simulink model "GVCU_HIL"  (R2026a)
settings: Solver=ode3  StartTime=0  StopTime=2474  FixedStep=0.0002
model workspace (MAT data in the model file):
  CANoelibParameters : object (value not decoded)
values from neighbouring files (symbols this model uses):
  acc_pedal_data = pedal_data.accelerator_pedal_position_t0    [Vehicle_Simulink_init.m]
  acc_pedal_time = pedal_data.t0    [Vehicle_Simulink_init.m]
  brk_pedal_data = brake_pedal_data.shared_brakes_drvrBrkPedlPerc_t0    [Vehicle_Simulink_init.m]
  brk_pedal_time = brake_pedal_data.t0    [Vehicle_Simulink_init.m]
  cycle_len = zeros(1, num_cycles)    [Vehicle_Simulink_init.m]
  cycle_speed_matrix = zeros(max_cycle_len, num_cycles)    [Vehicle_Simulink_init.m]
  cycle_time_matrix = zeros(max_cycle_len, num_cycles)    [Vehicle_Simulink_init.m]
  veh_speed_data = speed_data.shared_dynamicsVso_vehVelLgt_t0    [Vehicle_Simulink_init.m]
  veh_speed_time = speed_data.t0    [Vehicle_Simulink_init.m]
undefined symbols (not defined in the file or in its folder): Active, AuxActive, bat, environment, FL_prs_voltage, FR_prs_voltage, pos, RL_prs_voltage, RR_prs_voltage, tir, veh, VGetRawValueFlag, Voltage, VT2816_1_Ch1, VT2816_1_Ch2, VT2816_1_Ch3, VT2816_1_Ch4, VT2816_3_Ch13, VT2816_3_Ch14, VT7101_1_Out2, VT7820_2_Channel1, VT7820_2_Channel2, VT7820_2_Channel3, VT7820_2_Channel4, VTS
libraries: canoelib x144, autolibsharedcoupling x21, autolibcoupling x9, autolibshared x5, simulink_extras x4, simulink x4, slpidlib x3, autolibshareddiff x3, autolibutils x1, autolibdatasheetbattery x1, autolibmappedmotor x1, sl_discontinuities x1
(part 9 of 9)

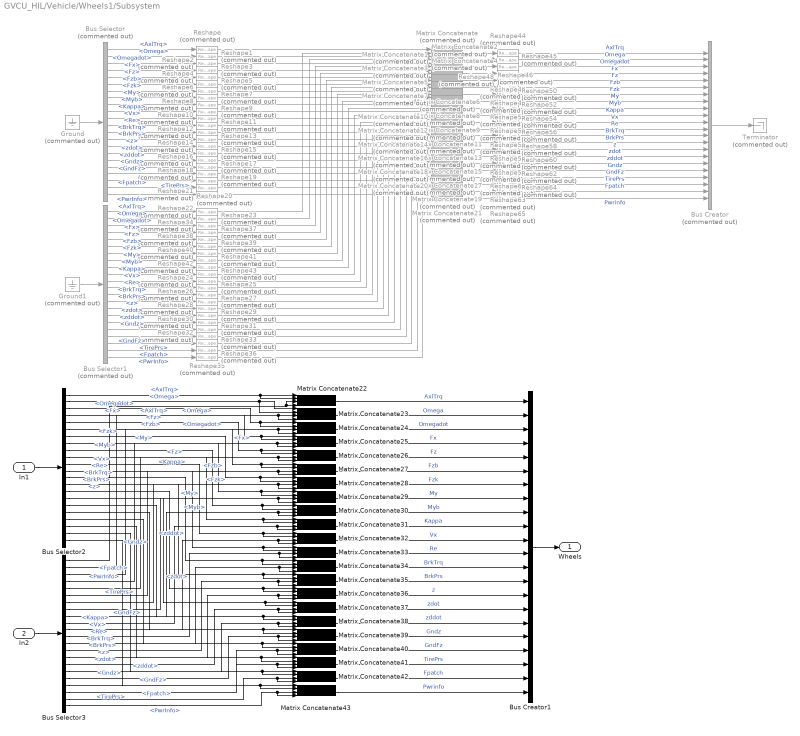
== system GVCU_HIL/Vehicle/Wheels1/Subsystem ==
  In1 : Inport
  In2 : Inport  Port=2
  Bus Creator : BusCreator  Commented=on  Inputs=22
  Bus Creator1 : BusCreator  Inputs=22
  Bus Selector : BusSelector  Commented=on  OutputSignals=AxlTrq,Omega,Omegadot,Fx,Fz,Fzb,Fzk,My,Myb,Kappa,Vx,Re,BrkTrq,BrkPrs,z,zdot,zddot,Gndz,GndFz,TirePrs,Fpatch,PwrInfo
  Bus Selector1 : BusSelector  Commented=on  OutputSignals=AxlTrq,Omega,Omegadot,Fx,Fz,Fzb,Fzk,My,Myb,Kappa,Vx,Re,BrkTrq,BrkPrs,z,zdot,zddot,Gndz,GndFz,TirePrs,Fpatch,PwrInfo
  Bus Selector2 : BusSelector  OutputSignals=AxlTrq,Omega,Omegadot,Fx,Fz,Fzb,Fzk,My,Myb,Kappa,Vx,Re,BrkTrq,BrkPrs,z,zdot,zddot,Gndz,GndFz,TirePrs,Fpatch,PwrInfo
  Bus Selector3 : BusSelector  OutputSignals=AxlTrq,Omega,Omegadot,Fx,Fz,Fzb,Fzk,My,Myb,Kappa,Vx,Re,BrkTrq,BrkPrs,z,zdot,zddot,Gndz,GndFz,TirePrs,Fpatch,PwrInfo
  Ground : Ground  Commented=on
  Ground1 : Ground  Commented=on
  Matrix Concatenate : Concatenate  Commented=on
  Matrix Concatenate{1..21} (21 alike) : Concatenate  Commented=on  ConcatenateDimension=2
  Matrix Concatenate{22..43} (22 alike) : Concatenate  NumInputs=4
  Reshape{,1..43} (44 alike) : Reshape  Commented=on  OutputDimensionality=Row vector (2-D)
  Reshape{44..65} (22 alike) : Reshape  Commented=on
  Terminator : Terminator  Commented=on
  Wheels : Outport
  wires:
  Bus Selector/1 -> Reshape/1  "<AxlTrq>"
  In2/1 -> Bus Selector3/1
  In1/1 -> Bus Selector2/1
  Bus Selector3/22 -> Matrix Concatenate43/3, Matrix Concatenate43/4  "<PwrInfo>"
  Bus Selector3/21 -> Matrix Concatenate42/3, Matrix Concatenate42/4  "<Fpatch>"
  Bus Selector3/20 -> Matrix Concatenate41/3, Matrix Concatenate41/4  "<TirePrs>"
  Bus Selector3/19 -> Matrix Concatenate40/3, Matrix Concatenate40/4  "<GndFz>"
  Bus Selector3/18 -> Matrix Concatenate39/3, Matrix Concatenate39/4  "<Gndz>"
  Bus Selector3/17 -> Matrix Concatenate38/3, Matrix Concatenate38/4  "<zddot>"
  Bus Selector3/16 -> Matrix Concatenate37/3, Matrix Concatenate37/4  "<zdot>"
  Bus Selector3/15 -> Matrix Concatenate36/3, Matrix Concatenate36/4  "<z>"
  Bus Selector3/14 -> Matrix Concatenate35/3, Matrix Concatenate35/4  "<BrkPrs>"
  Bus Selector3/13 -> Matrix Concatenate34/3, Matrix Concatenate34/4  "<BrkTrq>"
  Bus Selector3/12 -> Matrix Concatenate33/3, Matrix Concatenate33/4  "<Re>"
  Bus Selector3/11 -> Matrix Concatenate32/3, Matrix Concatenate32/4  "<Vx>"
  Bus Selector3/10 -> Matrix Concatenate31/3, Matrix Concatenate31/4  "<Kappa>"
  Bus Selector3/9 -> Matrix Concatenate30/3, Matrix Concatenate30/4  "<Myb>"
  Bus Selector3/8 -> Matrix Concatenate29/3, Matrix Concatenate29/4  "<My>"
  Bus Selector3/7 -> Matrix Concatenate28/3, Matrix Concatenate28/4  "<Fzk>"
  Bus Selector3/6 -> Matrix Concatenate27/3, Matrix Concatenate27/4  "<Fzb>"
  Bus Selector3/5 -> Matrix Concatenate26/3, Matrix Concatenate26/4  "<Fz>"
  Bus Selector3/4 -> Matrix Concatenate25/3, Matrix Concatenate25/4  "<Fx>"
  Bus Selector3/3 -> Matrix Concatenate24/3, Matrix Concatenate24/4  "<Omegadot>"
  Bus Selector3/2 -> Matrix Concatenate23/3, Matrix Concatenate23/4  "<Omega>"
  Bus Selector3/1 -> Matrix Concatenate22/3, Matrix Concatenate22/4  "<AxlTrq>"
  Matrix Concatenate23/1 -> Bus Creator1/2  "Omega"
  Matrix Concatenate29/1 -> Bus Creator1/8  "My"
  Matrix Concatenate36/1 -> Bus Creator1/15  "z"
  Matrix Concatenate27/1 -> Bus Creator1/6  "Fzb"
  Matrix Concatenate25/1 -> Bus Creator1/4  "Fx"
  Matrix Concatenate33/1 -> Bus Creator1/12  "Re"
  Matrix Concatenate28/1 -> Bus Creator1/7  "Fzk"
  Matrix Concatenate30/1 -> Bus Creator1/9  "Myb"
  Matrix Concatenate31/1 -> Bus Creator1/10  "Kappa"
  Matrix Concatenate43/1 -> Bus Creator1/22  "Pwrinfo"
  Matrix Concatenate22/1 -> Bus Creator1/1  "AxlTrq"
  Matrix Concatenate38/1 -> Bus Creator1/17  "zddot"
  Matrix Concatenate37/1 -> Bus Creator1/16  "zdot"
  Matrix Concatenate41/1 -> Bus Creator1/20  "TirePrs"
  Matrix Concatenate39/1 -> Bus Creator1/18  "Gndz"
  Matrix Concatenate24/1 -> Bus Creator1/3  "Omegadot"
  Matrix Concatenate26/1 -> Bus Creator1/5  "Fz"
  Matrix Concatenate35/1 -> Bus Creator1/14  "BrkPrs"
  Matrix Concatenate42/1 -> Bus Creator1/21  "Fpatch"
  Matrix Concatenate40/1 -> Bus Creator1/19  "GndFz"
  Matrix Concatenate34/1 -> Bus Creator1/13  "BrkTrq"
  Matrix Concatenate32/1 -> Bus Creator1/11  "Vx"
  Bus Creator1/1 -> Wheels/1
  Bus Selector2/22 -> Matrix Concatenate43/2, Matrix Concatenate43/1  "<PwrInfo>"
  Bus Selector2/21 -> Matrix Concatenate42/1, Matrix Concatenate42/2  "<Fpatch>"
  Bus Selector2/20 -> Matrix Concatenate41/1, Matrix Concatenate41/2  "<TirePrs>"
  Bus Selector2/19 -> Matrix Concatenate40/1, Matrix Concatenate40/2  "<GndFz>"
  Bus Selector2/18 -> Matrix Concatenate39/1, Matrix Concatenate39/2  "<Gndz>"
  Bus Selector2/17 -> Matrix Concatenate38/1, Matrix Concatenate38/2  "<zddot>"
  Bus Selector2/16 -> Matrix Concatenate37/1, Matrix Concatenate37/2  "<zdot>"
  Bus Selector2/15 -> Matrix Concatenate36/1, Matrix Concatenate36/2  "<z>"
  Bus Selector2/14 -> Matrix Concatenate35/1, Matrix Concatenate35/2  "<BrkPrs>"
  Bus Selector2/13 -> Matrix Concatenate34/2, Matrix Concatenate34/1  "<BrkTrq>"
  Bus Selector2/12 -> Matrix Concatenate33/1, Matrix Concatenate33/2  "<Re>"
  Bus Selector2/11 -> Matrix Concatenate32/2, Matrix Concatenate32/1  "<Vx>"
  Bus Selector2/10 -> Matrix Concatenate31/1, Matrix Concatenate31/2  "<Kappa>"
  Bus Selector2/9 -> Matrix Concatenate30/1, Matrix Concatenate30/2  "<Myb>"
  Bus Selector2/8 -> Matrix Concatenate29/1, Matrix Concatenate29/2  "<My>"
  Bus Selector2/7 -> Matrix Concatenate28/1, Matrix Concatenate28/2  "<Fzk>"
  Bus Selector2/6 -> Matrix Concatenate27/1, Matrix Concatenate27/2  "<Fzb>"
  Bus Selector2/5 -> Matrix Concatenate26/1, Matrix Concatenate26/2  "<Fz>"
  Bus Selector2/4 -> Matrix Concatenate25/1, Matrix Concatenate25/2  "<Fx>"
  Bus Selector2/3 -> Matrix Concatenate24/2, Matrix Concatenate24/1  "<Omegadot>"
  Bus Selector2/2 -> Matrix Concatenate23/2, Matrix Concatenate23/1  "<Omega>"
  Bus Selector2/1 -> Matrix Concatenate22/1, Matrix Concatenate22/2  "<AxlTrq>"
  Bus Creator/1 -> Terminator/1
  Reshape56/1 -> Bus Creator/13  "BrkTrq"
  Reshape54/1 -> Bus Creator/11  "Vx"
  Reshape55/1 -> Bus Creator/12  "Re"
  Reshape57/1 -> Bus Creator/14  "BrkPrs"
  Reshape58/1 -> Bus Creator/15  "z"
  Reshape59/1 -> Bus Creator/16  "zdot"
  Reshape60/1 -> Bus Creator/17  "zddot"
  Reshape61/1 -> Bus Creator/18  "Gndz"
  Reshape62/1 -> Bus Creator/19  "GndFz"
  Reshape63/1 -> Bus Creator/20  "TirePrs"
  Reshape64/1 -> Bus Creator/21  "Fpatch"
  Reshape65/1 -> Bus Creator/22  "Pwrinfo"
  Reshape53/1 -> Bus Creator/10  "Kappa"
  Reshape52/1 -> Bus Creator/9  "Myb"
  Reshape51/1 -> Bus Creator/8  "My"
  Reshape50/1 -> Bus Creator/7  "Fzk"
  Reshape49/1 -> Bus Creator/6  "Fzb"
  Reshape48/1 -> Bus Creator/5  "Fz"
  Reshape47/1 -> Bus Creator/4  "Fx"
  Reshape46/1 -> Bus Creator/3  "Omegadot"
  Reshape45/1 -> Bus Creator/2  "Omega"
  Reshape44/1 -> Bus Creator/1  "AxlTrq"
  Matrix Concatenate21/1 -> Reshape65/1
  Matrix Concatenate20/1 -> Reshape64/1
  Matrix Concatenate19/1 -> Reshape63/1
  Matrix Concatenate18/1 -> Reshape62/1
  Matrix Concatenate17/1 -> Reshape61/1
  Matrix Concatenate16/1 -> Reshape60/1
  Matrix Concatenate15/1 -> Reshape59/1
  Matrix Concatenate14/1 -> Reshape58/1
  Matrix Concatenate13/1 -> Reshape57/1
  Matrix Concatenate12/1 -> Reshape56/1
  Matrix Concatenate11/1 -> Reshape55/1
  Matrix Concatenate10/1 -> Reshape54/1
  Matrix Concatenate9/1 -> Reshape53/1
  Matrix Concatenate8/1 -> Reshape52/1
  Matrix Concatenate7/1 -> Reshape51/1
  Matrix Concatenate6/1 -> Reshape50/1
  Matrix Concatenate5/1 -> Reshape49/1
  Matrix Concatenate4/1 -> Reshape48/1
  Matrix Concatenate3/1 -> Reshape47/1
  Matrix Concatenate2/1 -> Reshape46/1
  Matrix Concatenate1/1 -> Reshape45/1
  Matrix Concatenate/1 -> Reshape44/1
  Reshape25/1 -> Matrix Concatenate11/2
  Reshape26/1 -> Matrix Concatenate12/2
  Reshape27/1 -> Matrix Concatenate13/2
  Reshape28/1 -> Matrix Concatenate14/2
  Reshape29/1 -> Matrix Concatenate15/2
  Reshape30/1 -> Matrix Concatenate16/2
  Reshape31/1 -> Matrix Concatenate17/2
  Reshape32/1 -> Matrix Concatenate18/2
  Reshape33/1 -> Matrix Concatenate19/2
  Reshape35/1 -> Matrix Concatenate20/2
  Reshape36/1 -> Matrix Concatenate21/2
  Reshape24/1 -> Matrix Concatenate10/2
  Reshape43/1 -> Matrix Concatenate9/2
  Reshape42/1 -> Matrix Concatenate8/2
  Reshape41/1 -> Matrix Concatenate7/2
  Reshape40/1 -> Matrix Concatenate6/2
  Reshape39/1 -> Matrix Concatenate5/2
  Reshape21/1 -> Matrix Concatenate21/1
  Reshape20/1 -> Matrix Concatenate20/1
  Reshape19/1 -> Matrix Concatenate19/1
  Reshape18/1 -> Matrix Concatenate18/1
  Reshape17/1 -> Matrix Concatenate17/1
  Reshape16/1 -> Matrix Concatenate16/1
  Reshape15/1 -> Matrix Concatenate15/1
  Reshape14/1 -> Matrix Concatenate14/1
  Reshape13/1 -> Matrix Concatenate13/1
  Reshape12/1 -> Matrix Concatenate12/1
  Reshape11/1 -> Matrix Concatenate11/1
  Reshape10/1 -> Matrix Concatenate10/1
  Reshape9/1 -> Matrix Concatenate9/1
  Reshape8/1 -> Matrix Concatenate8/1
  Reshape7/1 -> Matrix Concatenate7/1
  Reshape6/1 -> Matrix Concatenate6/1
  Reshape5/1 -> Matrix Concatenate5/1
  Reshape38/1 -> Matrix Concatenate4/2
  Reshape37/1 -> Matrix Concatenate3/2
  Reshape4/1 -> Matrix Concatenate4/1
  Reshape3/1 -> Matrix Concatenate3/1
  Reshape34/1 -> Matrix Concatenate2/2
  Reshape2/1 -> Matrix Concatenate2/1
  Reshape23/1 -> Matrix Concatenate1/2
  Reshape1/1 -> Matrix Concatenate1/1
  Reshape22/1 -> Matrix Concatenate/2
  Reshape/1 -> Matrix Concatenate/1
  Bus Selector1/19 -> Reshape32/1  "<GndFz>"
  Bus Selector1/13 -> Reshape26/1  "<BrkTrq>"
  Bus Selector1/15 -> Reshape28/1  "<z>"
  Bus Selector1/5 -> Reshape38/1  "<Fz>"
  Ground1/1 -> Bus Selector1/1
  Bus Selector1/14 -> Reshape27/1  "<BrkPrs>"
  Bus Selector1/1 -> Reshape22/1  "<AxlTrq>"
  Bus Selector1/10 -> Reshape43/1  "<Kappa>"
  Bus Selector1/6 -> Reshape39/1  "<Fzb>"
  Bus Selector1/11 -> Reshape24/1  "<Vx>"
  Bus Selector1/18 -> Reshape31/1  "<Gndz>"
  Bus Selector1/8 -> Reshape41/1  "<My>"
  Bus Selector1/22 -> Reshape36/1  "<PwrInfo>"
  Bus Selector1/21 -> Reshape35/1  "<Fpatch>"
  Bus Selector1/17 -> Reshape30/1  "<zddot>"
  Bus Selector1/2 -> Reshape23/1  "<Omega>"
  Bus Selector1/12 -> Reshape25/1  "<Re>"
  Bus Selector1/20 -> Reshape33/1  "<TirePrs>"
  Bus Selector1/9 -> Reshape42/1  "<Myb>"
  Bus Selector1/16 -> Reshape29/1  "<zdot>"
  Bus Selector1/7 -> Reshape40/1  "<Fzk>"
  Bus Selector1/3 -> Reshape34/1  "<Omegadot>"
  Bus Selector1/4 -> Reshape37/1  "<Fx>"
  Bus Selector/22 -> Reshape21/1  "<PwrInfo>"
  Bus Selector/21 -> Reshape20/1  "<Fpatch>"
  Bus Selector/20 -> Reshape19/1  "<TirePrs>"
  Bus Selector/19 -> Reshape18/1  "<GndFz>"
  Bus Selector/18 -> Reshape17/1  "<Gndz>"
  Bus Selector/17 -> Reshape16/1  "<zddot>"
  Bus Selector/16 -> Reshape15/1  "<zdot>"
  Bus Selector/15 -> Reshape14/1  "<z>"
  Bus Selector/14 -> Reshape13/1  "<BrkPrs>"
  Bus Selector/13 -> Reshape12/1  "<BrkTrq>"
  Bus Selector/12 -> Reshape11/1  "<Re>"
  Bus Selector/11 -> Reshape10/1  "<Vx>"
  Bus Selector/10 -> Reshape9/1  "<Kappa>"
  Bus Selector/9 -> Reshape8/1  "<Myb>"
  Bus Selector/8 -> Reshape7/1  "<My>"
  Bus Selector/7 -> Reshape6/1  "<Fzk>"
  Bus Selector/6 -> Reshape5/1  "<Fzb>"
  Bus Selector/5 -> Reshape4/1  "<Fz>"
  Bus Selector/4 -> Reshape3/1  "<Fx>"
  Bus Selector/3 -> Reshape2/1  "<Omegadot>"
  Bus Selector/2 -> Reshape1/1  "<Omega>"
  Ground/1 -> Bus Selector/1

== system GVCU_HIL/Vehicle/Wheels1/whel to axel transform3 ==
  Input (1x4) : Inport
  Selector4 : Selector  InputPortWidth=4  IndexOptions=Index vector (dialog)  Indices=[1]  OutputSizes=1
  Selector5 : Selector  InputPortWidth=4  IndexOptions=Index vector (dialog)  Indices=[2]  OutputSizes=1
  Selector6 : Selector  InputPortWidth=4  IndexOptions=Index vector (dialog)  Indices=[3]  OutputSizes=1
  Selector7 : Selector  InputPortWidth=4  IndexOptions=Index vector (dialog)  Indices=[4]  OutputSizes=1
  "Front L " : Outport
  Front R : Outport  Port=2
  "Rear L " : Outport  Port=3
  Rear R : Outport  Port=4
  wires:
  Selector7/1 -> Rear R/1
  Selector6/1 -> "Rear L "/1
  Selector5/1 -> Front R/1
  Selector4/1 -> "Front L "/1
  Input (1x4)/1 -> Selector4/1, Selector5/1, Selector7/1, Selector6/1

== matlab function GVCU_HIL/Clutch handling/Offset_substraction/MATLAB Function ==
  data: drvMode input; y output; pPa input
function y = fcn(drvMode, pPa)
% drvMode : drive mode input
% pPa     : measured pressure input in Pa
% y       : pressure output with learned offset removed, in Pa

persistent prevDrvMode state timer sumP sampleCount offset

if isempty(prevDrvMode)
    prevDrvMode = drvMode;
    state = uint8(0);      % 0=idle, 1=wait, 2=average, 3=hold
    timer = 0.0;
    sumP = 0.0;
    sampleCount = uint32(0);
    offset = 0.0;
end

T = 0.0002;          % sample time [s]
WAIT_TIME = 0.5;     % wait time after drvMode becomes 1 [s]
AVG_TIME  = 0.2;     % averaging time [s]
ONE_BAR_PA = 1e5;    % 1 bar in Pa

% Trigger when drvMode becomes 1, regardless of previous value
if (prevDrvMode ~= 1) && (drvMode == 1)
    state = uint8(1);
    timer = 0.0;
    sumP = 0.0;
    sampleCount = uint32(0);
end

switch state
    case 0
        % Idle state

    case 1
        % Wait for 0.5 s
        timer = timer + T;
        if timer >= WAIT_TIME
            state = uint8(2);
            timer = 0.0;
            sumP = 0.0;
            sampleCount = uint32(0);
        end

    case 2
        % Average pressure for 0.2 s
        timer = timer + T;
        sumP = sumP + pPa;
        sampleCount = sampleCount + 1;

        if timer >= AVG_TIME
            if sampleCount > 0
                offset = sumP / double(sampleCount) - ONE_BAR_PA;
            else
                offset = 0.0;
            end
            state = uint8(3);
        end

    case 3
        % Hold learned offset
end

% Output compensated pressure
y = pPa - offset;

prevDrvMode = drvMode;

== matlab function GVCU_HIL/Powertrain (EV)/PID Speed Ctrl Mode/MATLAB Function1 ==
  settings: updateMethod=DISCRETE
  data: spdErr_rads input; trq_cmd output; trq_fwd input; trq_act input; lim_pos input; lim_neg input; reset input
function trq_cmd = speedPID(spdErr_rads, trq_fwd, trq_act, lim_pos, lim_neg, reset)
%#codegen
% Speed PID + feedforward, output clamped.
% Replicates inverter torque_handler.c trqHandlerSpeedCtrl()
%
% Inputs:
%   spdErr_rads  [rad/s]   speed error (spd_req - spd_fb), computed externally
%   trq_fwd      [Nm]      feedforward torque = GVCU torque request (added internally)
%   trq_act      [Nm]      actual motor torque feedback (e.g. EM_trq from motor model)
%   lim_pos      [Nm]      upper output clamp
%   lim_neg      [Nm]      lower output clamp
%   reset                  from spdCtrlReset block (>0.5 = active)
%
% Output:
%   trq_cmd  [Nm]      clamped torque command (PID + feedforward)
%
% Gains (caldata.c index 0, RPM-based, Ts=500us):
%   kp=2.5, ki=0.004, kaw=0.0035, kd=0

persistent intgl trqReqPrev

if isempty(intgl)
    intgl      = 0;
    trqReqPrev = 0;
end

Ts      = 0.0002;       % actual Simulink step size
Ts_inv  = 0.0005;       % inverter design step size
scale   = Ts / Ts_inv;  % = 0.4

% values from Set 3 
kp  = 2; %0.78;
ki  = 0.035 * scale;    % = 0.0016
kaw = 0.005 * scale;   % = 0.0014

if reset > 0.5
    intgl      = 0;
    trqReqPrev = 0;
    trq_cmd    = 0;
    return;
end

% Speed error in RPM (matches inverter: spdErr = spdReq - ctrlOutSpeed)
spdErr = spdErr_rads * (60 / (2*pi));

% Integrator update with anti-windup
% Matches inverter: spdIntgl += ki*spdErr + kaw*(trqAct - trqReq_prev_unclamped)
intgl = intgl + ki * spdErr + kaw * (trq_act - trqReqPrev);

% Unclamped total output (PID + feedforward)
trq_req_unc = kp * spdErr + intgl + trq_fwd;

% Clamp output
trq_cmd = max(lim_neg, min(lim_pos, trq_req_unc));

% Store unclamped total for next step's anti-windup
trqReqPrev = trq_cmd;

== matlab function GVCU_HIL/Brake_HIL/Simulated GVCU - Steering /MATLAB Function1 ==
  settings: updateMethod=DISCRETE  sampleTime=0.1
  data: y output
function y = counterFcn()
    persistent count;
    if isempty(count)
        count = 0; % Initialize counter
    end
    count = mod(count + 1, 15); % 4-bit counter (0-15)
    y = count; % Use uint8 to avoid Fixed-Point Designer
end

== matlab function GVCU_HIL/Powertrain (EV)/PID Speed Controller/MATLAB Function ==
  settings: updateMethod=DISCRETE
  data: EM_Spd input; reset_out output; speed_req input; t input
function reset_out = spdCtrlReset(EM_Spd, speed_req, t)
% Resets PID integrator when both speeds are below threshold for 500ms.
% Matches real inverter: cInvStopSpeed = 20 RPM, SPD_CTRL_RESET_DELAY = 500ms
% Input t: simulation time from Clock block [s]

persistent stop_ts fired

if isempty(stop_ts)
    stop_ts = 0;
    fired   = false;
end

SPD_THRESHOLD  = 2.094;  % 20 RPM in rad/s  (= cInvStopSpeed)
RESET_DELAY_S  = 0.5;    % 500ms in s       (= SPD_CTRL_RESET_DELAY)

if (abs(EM_Spd) < SPD_THRESHOLD) && (abs(speed_req) < SPD_THRESHOLD)
    if stop_ts == 0
        stop_ts = t;     % Start timer: record entry time
    end

    if ((t - stop_ts) >= RESET_DELAY_S) && (~fired)
        reset_out = 1.0; % Rising edge -> reset PID integrator
        fired     = true;
    else
        reset_out = 0.0;
    end
else
    stop_ts   = 0;       % Reset timer
    fired     = false;   % Allow trigger again next standstill
    reset_out = 0.0;
end

== matlab function GVCU_HIL/Brake_HIL/Simulated GVCU - Steering /MATLAB Function2 ==
  data: switch_state input; drv_st output
function drv_st   = update_drv_st(switch_state)
    % Persistent variables to maintain state across function calls
    persistent drv_st_internal last_switch_state last_update_time;
    
    if isempty(drv_st_internal)
        drv_st_internal = 1;  % Initial state of drv_st
        last_switch_state = 0; % Initial switch state
        last_update_time = tic; % Start timer
    end
    
    if switch_state == 1
        
        if last_switch_state == 0
            % Switch was just turned ON, reset timer and set drv_st to 1
            drv_st_internal = 1;
            last_update_time = tic;
        else
            % Check elapsed time since last update
            elapsed_time = toc(last_update_time);
            if drv_st_internal == 1 && elapsed_time >= 2
                drv_st_internal = 2;
                last_update_time = tic;
            elseif drv_st_internal == 2 && elapsed_time >= 2
                drv_st_internal = 4;
                last_update_time = tic;
            end
        end
        
    else
        
        drv_st_internal = 1; % Reset drv_st if switch is OFF
    end
    
    last_switch_state = switch_state; % Update switch state memory
    drv_st = drv_st_internal; % Output the updated drv_st value
end

== matlab function GVCU_HIL/Brake_HIL/Simulated GVCU - Steering /MATLAB Function3 ==
  settings: updateMethod=DISCRETE  sampleTime=0.01
  data: y output
function y = counterFcn()
    persistent count;
    if isempty(count)
        count = 0; % Initialize counter
    end
    count = mod(count + 1, 15); % 4-bit counter (0-15)
    y = count; % Use uint8 to avoid Fixed-Point Designer
end

== matlab function GVCU_HIL/Brake_HIL/Simulated GVCU - Steering /MATLAB Function4 ==
  settings: updateMethod=DISCRETE  sampleTime=0.01
  data: y output
function y = counterFcn()
    persistent count;
    if isempty(count)
        count = 0; % Initialize counter
    end
    count = mod(count + 1, 15); % 4-bit counter (0-15)
    y = count; % Use uint8 to avoid Fixed-Point Designer
end

== matlab function GVCU_HIL/Brake_HIL/Simulated GVCU - Steering /MATLAB Function5 ==
  settings: updateMethod=DISCRETE  sampleTime=0.1
  data: y output
function y = counterFcn()
    persistent count;
    if isempty(count)
        count = 0; % Initialize counter
    end
    count = mod(count + 1, 15); % 4-bit counter (0-15)
    y = count; % Use uint8 to avoid Fixed-Point Designer
end

== matlab function GVCU_HIL/Inverter/INV ==
  data: inv_st_prev input; inv_st output; inv_ena_req input; motor_ena_req input; inv_shutdown_req input
function inv_st = fcn(inv_st_prev, inv_ena_req, motor_ena_req, inv_shutdown_req)
	switch inv_st_prev
		case 0
			if (1 == inv_ena_req)
				inv_st_local = 1;
			else
				inv_st_local = 0;
			end
		case 1
			if (1 == inv_ena_req)
				inv_st_local = 2;
			else
				inv_st_local = 0;
			end	
		case 2
			if (1 == inv_ena_req)
				inv_st_local = 3;
			else
				inv_st_local = 0;
			end
		case 3
			if ((1 == inv_ena_req) && (1 == motor_ena_req))
				inv_st_local = 4;
			else
				inv_st_local = 3;
			end
		case 4
			if ((1 ~= inv_ena_req) || (1 ~= motor_ena_req) || (1 == inv_shutdown_req))
				inv_st_local = 0;
			else
				inv_st_local = 4;
			end
		case 5
			inv_st_local = 0;
		case 6
			inv_st_local = 0;
		otherwise
			inv_st_local = 0;
	end
	inv_st = inv_st_local;
 
end

== matlab function GVCU_HIL/GVCU - HiL/BMS ==
  data: bms_st_prev input; pwr_st input; bms_st output; hyb_st input
function bms_st = fcn(bms_st_prev, pwr_st, hyb_st)
	switch bms_st_prev
		case 0
			bms_st_local = 5;
		case 1
			if (7 ~= pwr_st)
				bms_st_local = 5;
            elseif (4 == hyb_st)
				bms_st_local = 3;
			else
				bms_st_local = 1;
			end	
		case 2
			bms_st_local = 5;
		case 3
			if (7 ~= pwr_st)
				bms_st_local = 5;
			else
				bms_st_local = 3;
			end
		case 4
			bms_st_local = 5;
		case 5
			if (7 == pwr_st)
				bms_st_local = 3;
			else
				bms_st_local = 5;
			end
		case 6
			bms_st_local = 5;
		otherwise
			bms_st_local = 5;
	end
    bms_st = bms_st_local;
end

== matlab function GVCU_HIL/Wheel_rates/MATLAB Function2 ==
  data: wheel_rate input; wheel_direction output
function wheel_direction = wheel_direction(wheel_rate)

STATIONARY_THD = 0.01; % rad/s
 
if abs(wheel_rate) <= STATIONARY_THD

    wheel_direction = 2; % STATIONARY

elseif wheel_rate > STATIONARY_THD

    wheel_direction = 3; % FORWARD

elseif wheel_rate < -STATIONARY_THD

    wheel_direction = 4; % REARWARD

else

    wheel_direction = 0; % UNKNOWN (NaN)

end

== matlab function GVCU_HIL/Driver/MATLAB Function ==
  settings: updateMethod=DISCRETE
  data: t_sim input; input_mode input; t_spd input; spd_data input; cycle_idx input; cycle_time_matrix input; cycle_speed_matrix input; cycle_len input; vel_ref input; vel_out output; cycle_time_remaining output; cycle_finished output
function [vel_out, cycle_time_remaining, cycle_finished] = fcn(t_sim, input_mode, t_spd, spd_data, ...
                                                              cycle_idx, cycle_time_matrix, cycle_speed_matrix, cycle_len, vel_ref)

persistent t_mode_start last_mode last_cycle;

if isempty(t_mode_start)
    t_mode_start = -1;
    last_mode    = 0;
    last_cycle   = 0;
end

% Default: WLTC3b
default_cycle_idx = 4;

% Safe cycle index
idx = round(cycle_idx);

if isnan(idx) || idx < 1 || idx > size(cycle_time_matrix, 2)
    idx = default_cycle_idx;
end

% Restart timing when mode changes to replay modes
if (input_mode == 2 || input_mode == 3) && last_mode ~= input_mode
    t_mode_start = t_sim;
end

% Restart drive cycle when selected cycle changes while input_mode == 3
if input_mode == 3 && last_cycle ~= idx
    t_mode_start = t_sim;
end

last_mode  = input_mode;
last_cycle = idx;

% Default outputs
vel_out              = vel_ref;
cycle_time_remaining = 0;
cycle_finished       = 0;

if input_mode == 2 && t_mode_start >= 0

    % Recorded speed replay
    t_rel = t_sim - t_mode_start;
    t_rel = min(t_rel, t_spd(end));

    vel_out = interp1(t_spd, spd_data, t_rel, 'linear', spd_data(end));

elseif input_mode == 3 && t_mode_start >= 0

    % Drive cycle replay
    n = int32(cycle_len(idx));

    cycle_end_time = cycle_time_matrix(n, idx);

    t_rel = t_sim - t_mode_start;

    % Remaining time of selected cycle
    cycle_time_remaining = max(cycle_end_time - t_rel, 0);

    if t_rel >= cycle_end_time
        cycle_finished = 1;
        t_rel = cycle_end_time;
    end

    cycle_time  = cycle_time_matrix(1:n, idx);
    cycle_speed = cycle_speed_matrix(1:n, idx);

    vel_out = interp1(cycle_time, cycle_speed, t_rel, 'linear', cycle_speed(end));

end

== matlab function GVCU_HIL/Driver/MATLAB Function2 ==
  settings: updateMethod=DISCRETE
  data: RefVel input; RefVel output; trans_park_neutral input; ign output; brake_switch output; btn_paddle_ri output; btn_paddle_le output; trans_neutral_drive input; trans_park_drive input
function [RefVel, ign, brake_switch, btn_paddle_ri, btn_paddle_le] = update_drv_st(RefVel, trans_park_neutral, trans_neutral_drive, trans_park_drive)
persistent main_state sub_state t_start
persistent brake_switch_internal
persistent btn_paddle_ri_internal btn_paddle_le_internal
persistent prev_trans_park_neutral prev_trans_neutral_drive prev_trans_park_drive
persistent pending_park_neutral pending_neutral_drive pending_park_drive

% main_state:
% 0 = idle
% 1 = Park -> Neutral
% 2 = Neutral -> Drive
% 3 = Park -> Drive
%
% signal convention:
% brake_switch: 1 = released, 2 = pressed
% btn_paddle_ri: 1 = released, 2 = pressed
% btn_paddle_le: 1 = released, 2 = pressed

if isempty(main_state)
    main_state = 0;
    sub_state = 0;
    t_start = tic;

    brake_switch_internal = 1;
    btn_paddle_ri_internal = 1;
    btn_paddle_le_internal = 1;

    prev_trans_park_neutral = 0;
    prev_trans_neutral_drive = 0;
    prev_trans_park_drive = 0;

    pending_park_neutral = 0;
    pending_neutral_drive = 0;
    pending_park_drive = 0;
end

ign = 7;
refVelInp = RefVel;

% Capture button rising edges and store as one-shot pending requests.
if trans_park_neutral && ~prev_trans_park_neutral
    pending_park_neutral = 1;
end
if trans_neutral_drive && ~prev_trans_neutral_drive
    pending_neutral_drive = 1;
end
if trans_park_drive && ~prev_trans_park_drive
    pending_park_drive = 1;
end

prev_trans_park_neutral = trans_park_neutral;
prev_trans_neutral_drive = trans_neutral_drive;
prev_trans_park_drive = trans_park_drive;

% Only start a new transition when no other transition is active
if main_state == 0
    if pending_park_drive
        main_state = 3;
        sub_state = 0;
        t_start = tic;
        pending_park_drive = 0;

    elseif pending_park_neutral
        main_state = 1;
        sub_state = 0;
        t_start = tic;
        pending_park_neutral = 0;

    elseif pending_neutral_drive
        main_state = 2;
        sub_state = 0;
        t_start = tic;
        pending_neutral_drive = 0;
    end
end

switch main_state
    case 0
        % Idle:
        % keep RefVel input
        % release buttons and brake
        RefVel = refVelInp;
        brake_switch_internal = 1;
        btn_paddle_ri_internal = 1;
        btn_paddle_le_internal = 1;

    case 1
        % Park -> Neutral
        % RefVel forced to zero during transition
        RefVel = 0;

        switch sub_state
            case 0
                % Press brake first
                brake_switch_internal = 2;
                btn_paddle_ri_internal = 1;
                btn_paddle_le_internal = 1;

                sub_state = 1;
                t_start = tic;

            case 1
                % Press both paddles for 1 second
                brake_switch_internal = 2;
                btn_paddle_ri_internal = 2;
                btn_paddle_le_internal = 2;

                if toc(t_start) >= 1.0
                    sub_state = 2;
                    t_start = tic;
                end

            case 2
                % Release both paddles, keep brake pressed
                brake_switch_internal = 2;
                btn_paddle_ri_internal = 1;
                btn_paddle_le_internal = 1;

                if toc(t_start) >= 0.2
                    sub_state = 3;
                end

            case 3
                % Finish in Neutral, then return to idle
                brake_switch_internal = 1;
                btn_paddle_ri_internal = 1;
                btn_paddle_le_internal = 1;

                main_state = 0;
                sub_state = 0;
        end

    case 2
        % Neutral -> Drive
        % RefVel forced to zero during transition
        RefVel = 0;

        switch sub_state
            case 0
                % Press brake first
                brake_switch_internal = 2;
                btn_paddle_ri_internal = 1;
                btn_paddle_le_internal = 1;

                sub_state = 1;
                t_start = tic;

            case 1
                % Press right paddle for 1 second
                brake_switch_internal = 2;
                btn_paddle_ri_internal = 2;
                btn_paddle_le_internal = 1;

                if toc(t_start) >= 1.0
                    sub_state = 2;
                    t_start = tic;
                end

            case 2
                % Release right paddle, keep brake pressed
                brake_switch_internal = 2;
                btn_paddle_ri_internal = 1;
                btn_paddle_le_internal = 1;

                if toc(t_start) >= 0.2
                    sub_state = 3;
                end

            case 3
                % Release brake after paddle release
                brake_switch_internal = 1;
                btn_paddle_ri_internal = 1;
                btn_paddle_le_internal = 1;

                main_state = 0;
                sub_state = 0;
        end

    case 3
        % Park -> Drive
        % RefVel forced to zero during transition
        RefVel = 0;

        switch sub_state
            case 0
                % Press brake first
                brake_switch_internal = 2;
                btn_paddle_ri_internal = 1;
                btn_paddle_le_internal = 1;

                sub_state = 1;
                t_start = tic;

            case 1
                % Press both paddles for 1 second
                brake_switch_internal = 2;
                btn_paddle_ri_internal = 2;
                btn_paddle_le_internal = 2;

                if toc(t_start) >= 1.0
                    sub_state = 2;
                    t_start = tic;
                end

            case 2
                % Release both paddles -> Neutral, keep brake pressed
                brake_switch_internal = 2;
                btn_paddle_ri_internal = 1;
                btn_paddle_le_internal = 1;

                if toc(t_start) >= 0.2
                    sub_state = 3;
                    t_start = tic;
                end

            case 3
                % Press right paddle for 1 second
                brake_switch_internal = 2;
                btn_paddle_ri_internal = 2;
                btn_paddle_le_internal = 1;

                if toc(t_start) >= 1.0
                    sub_state = 4;
                    t_start = tic;
                end

            case 4
                % Release right paddle -> Drive, keep brake pressed
                brake_switch_internal = 2;
                btn_paddle_ri_internal = 1;
                btn_paddle_le_internal = 1;

                if toc(t_start) >= 0.2
                    sub_state = 5;
                end

            case 5
                % Release brake
                brake_switch_internal = 1;
                btn_paddle_ri_internal = 1;
                btn_paddle_le_internal = 1;

                main_state = 0;
                sub_state = 0;
        end
end

% Assign outputs from persistent internal values
brake_switch = brake_switch_internal;
btn_paddle_ri = btn_paddle_ri_internal;
btn_paddle_le = btn_paddle_le_internal;

== matlab function GVCU_HIL/Driver/MATLAB Function1 ==
  settings: updateMethod=DISCRETE
  data: t_sim input; input_mode input; t_pedal input; pedal_data input; acc_pedal_drvr input; brk_pedal_drvr input; t_brake input; pedal_out output; brake_data input; brake_out output
function [pedal_out, brake_out] = fcn(t_sim, input_mode, t_pedal, pedal_data, acc_pedal_drvr, brk_pedal_drvr, t_brake, brake_data)
persistent t_mode_start last_mode;

if isempty(t_mode_start)
    t_mode_start = -1;
    last_mode    = 0;
end

if input_mode == 1 && last_mode ~= 1
    t_mode_start = t_sim;
end
last_mode = input_mode;

if input_mode == 1 && t_mode_start >= 0
    t_rel     = t_sim - t_mode_start;
    pedal_out = interp1(t_pedal, pedal_data, min(t_rel, t_pedal(end)), 'linear', pedal_data(end));
    brake_out = interp1(t_brake, brake_data, min(t_rel, t_brake(end)), 'linear', brake_data(end));
else
    pedal_out = acc_pedal_drvr;
    brake_out = brk_pedal_drvr;
end

== matlab function GVCU_HIL/Powertrain (EV)/PID Speed Ctrl Mode/MATLAB Function ==
  settings: updateMethod=DISCRETE
  data: EM_Spd input; reset_out output; speed_req input; t input
function reset_out = spdCtrlReset(EM_Spd, speed_req, t)
% Resets PID integrator when both speeds are below threshold for 500ms.
% Matches real inverter: cInvStopSpeed = 20 RPM, SPD_CTRL_RESET_DELAY = 500ms
% Input t: simulation time from Clock block [s]

persistent stop_ts fired

if isempty(stop_ts)
    stop_ts = 0;
    fired   = false;
end

SPD_THRESHOLD  = 2.094;  % 20 RPM in rad/s  (= cInvStopSpeed)
RESET_DELAY_S  = 0.5;    % 500ms in s       (= SPD_CTRL_RESET_DELAY)

if (abs(EM_Spd) < SPD_THRESHOLD) && (abs(speed_req) < SPD_THRESHOLD)
    if stop_ts == 0
        stop_ts = t;     % Start timer: record entry time
    end

    if ((t - stop_ts) >= RESET_DELAY_S) && (~fired)
        reset_out = 1.0; % Rising edge -> reset PID integrator
        fired     = true;
    else
        reset_out = 0.0;
    end
else
    stop_ts   = 0;       % Reset timer
    fired     = false;   % Allow trigger again next standstill
    reset_out = 0.0;
end
